simulink library "gravityGrad_Lib"  (R2018b)
settings: Solver=VariableStepAuto  StartTime=0.0  StopTime=10.0  RelTol=1e-3
undefined symbols (not defined in the file or in its folder): fswParams, simParams
libraries: vrlib x4, aerolibutil x1, aerolibgravity2 x1
settings Model: Creator=im11  LastModifiedBy=Taylor

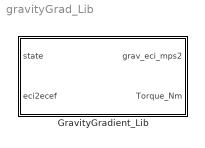
== system gravityGrad_Lib ==
  "GravityGradient_Lib " : Subsystem

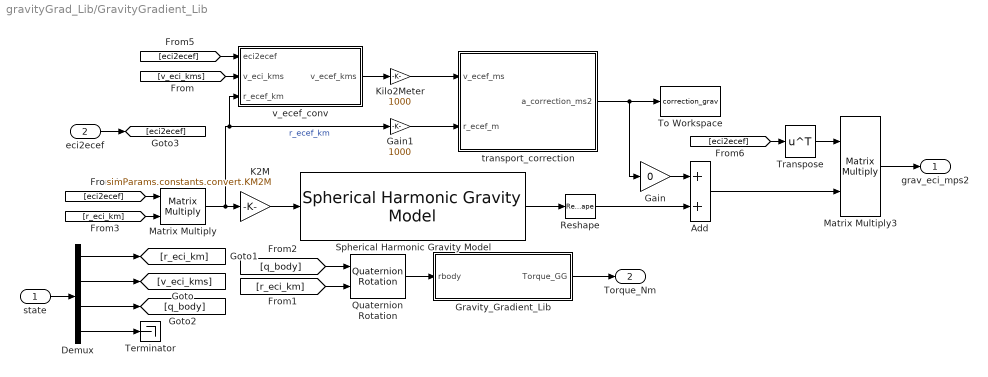
== system gravityGrad_Lib/GravityGradient_Lib  ==
  state : Inport
  "eci2ecef " : Inport  Port=2
  Add : Sum
  Demux : Demux  Outputs=[3 3 4 3]
  Gain : Gain  Gain=0
  Gain1 : Gain  Gain=1000
  "Gravity_Gradient_Lib " : MATLAB Function  TreatAsAtomicUnit=on
  "K2M " : Gain  Gain=simParams.constants.convert.KM2M
  "Kilo2Meter " : Gain  Gain=1000
  Matrix Multiply : Product  Multiplication=Matrix(*)
  Matrix Multiply3 : Product  Multiplication=Matrix(*)
  Quaternion Rotation : aerolibutil/Quaternion Rotation
  Reshape : Reshape  OutputDimensionality=Customize  OutputDimensions=3
  Spherical Harmonic Gravity Model : aerolibgravity2/Spherical Harmonic Gravity Model  units=Metric (MKS)  degree=40  action=Warning  ptype=EGM2008  datafile='aerogmm2b.mat'
      settings: SourceProductName=Aerospace Blockset  SourceProductBaseCode=AE
  Terminator : Terminator
  To Workspace : ToWorkspace  VariableName=correction_grav  SaveFormat=Timeseries  SampleTime=-1
  Transpose : Math  Operator=transpose  SaturateOnIntegerOverflow=on
  transport_correction : Subsystem
  v_ecef_conv : Subsystem
  grav_eci_mps2 : Outport
  Torque_Nm : Outport  Port=2
  wires:
  "Gravity_Gradient_Lib "/1(Torque_GG) -> Torque_Nm/1
  "K2M "/1 -> Spherical Harmonic Gravity Model/1
  [eci2ecef] -> v_ecef_conv/1(eci2ecef)
  v_ecef_conv/1(v_ecef_kms) -> "Kilo2Meter "/1
  [r_eci_km] -> Quaternion Rotation/2
  [v_eci_kms] -> v_ecef_conv/2(v_eci_kms)
  "eci2ecef "/1 -> [eci2ecef]
  Matrix Multiply3/1 -> grav_eci_mps2/1
  Demux/2 -> [v_eci_kms]
  [eci2ecef] -> Transpose/1
  [q_body] -> Quaternion Rotation/1
  [eci2ecef] -> Matrix Multiply/1
  Quaternion Rotation/1 -> "Gravity_Gradient_Lib "/1(rbody)
  Transpose/1 -> Matrix Multiply3/1
  state/1 -> Demux/1
  Demux/1 -> [r_eci_km]
  "Kilo2Meter "/1 -> transport_correction/1(v_ecef_ms)
  Gain1/1 -> transport_correction/2(r_ecef_m)
  Demux/4 -> Terminator/1
  [r_eci_km] -> Matrix Multiply/2
  Demux/3 -> [q_body]
  Matrix Multiply/1 -> Gain1/1, v_ecef_conv/3(r_ecef_km), "K2M "/1  "r_ecef_km"
  transport_correction/1(a_correction_ms2) -> To Workspace/1, Gain/1
  Reshape/1 -> Add/2
  Spherical Harmonic Gravity Model/1 -> Reshape/1
  Add/1 -> Matrix Multiply3/2
  Gain/1 -> Add/1

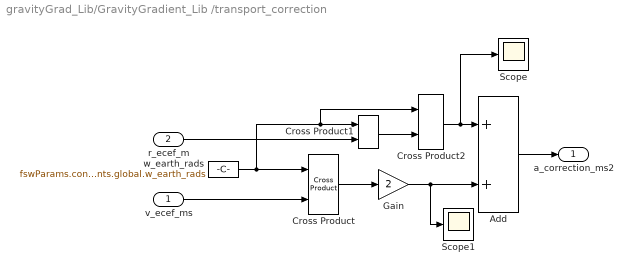
== system gravityGrad_Lib/GravityGradient_Lib /transport_correction ==
  v_ecef_ms : Inport
  r_ecef_m : Inport  Port=2
  Add : Sum
  Cross Product : vrlib/Utilities/Cross Product
      settings: SourceProductBaseCode=VR
  Cross Product1 : vrlib/Utilities/Cross Product
      settings: SourceProductBaseCode=VR
  Cross Product2 : vrlib/Utilities/Cross Product
      settings: SourceProductBaseCode=VR
  Gain : Gain  Gain=2
  Scope : Scope
  Scope1 : Scope
  w_earth_rads : Constant  Value=fswParams.constants.global.w_earth_rads
  a_correction_ms2 : Outport
  wires:
  Gain/1 -> Add/2, Scope1/1
  Add/1 -> a_correction_ms2/1
  w_earth_rads/1 -> Cross Product1/1, Cross Product2/1, Cross Product/1
  Cross Product1/1 -> Cross Product2/2
  r_ecef_m/1 -> Cross Product1/2
  v_ecef_ms/1 -> Cross Product/2
  Cross Product/1 -> Gain/1
  Cross Product2/1 -> Add/1, Scope/1

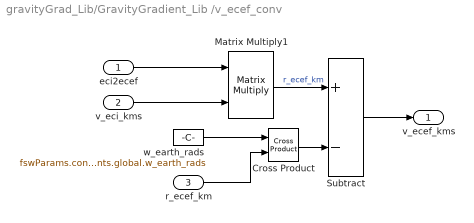
== system gravityGrad_Lib/GravityGradient_Lib /v_ecef_conv ==
  eci2ecef : Inport
  v_eci_kms : Inport  Port=2
  r_ecef_km : Inport  Port=3
  Cross Product : vrlib/Utilities/Cross Product
      settings: SourceProductBaseCode=VR
  Matrix Multiply1 : Product  Multiplication=Matrix(*)
  Subtract : Sum  Inputs=+-
  w_earth_rads : Constant  Value=fswParams.constants.global.w_earth_rads
  v_ecef_kms : Outport
  wires:
  w_earth_rads/1 -> Cross Product/1
  v_eci_kms/1 -> Matrix Multiply1/2
  eci2ecef/1 -> Matrix Multiply1/1
  Cross Product/1 -> Subtract/2
  Subtract/1 -> v_ecef_kms/1
  r_ecef_km/1 -> Cross Product/2
  Matrix Multiply1/1 -> Subtract/1  "r_ecef_km"

== matlab function gravityGrad_Lib/GravityGradient_Lib /Gravity_Gradient_Lib  ==
  data: rbody input; Torque_GG output; simParams parameter
function Torque_GG   = GravityG(rbody,simParams)
%r_body is the position vector in the body frame of the CubeSat
%J is the moment of inertia
%q is the unit quaternion 
%This will output the gravity gradient torques from the initial position

J = simParams.scParams.J;

rbody = rbody*1000; %converting to meters

mu = 3.986004418e14; % in m^3/s^2
Ro = sqrt(rbody(1)^2+rbody(2)^2+rbody(3)^2);%in meters
L = 30e-2;%Longest length of CubeSat in meters

a   = rbody;
b   = J*rbody;
axb = skew(a)*b;

Torque_GG = 3*mu/(norm(a)^5)*axb;%N-m %Gravity Gradient Torques
%Force_GG = Torque_GG/L; %N


end
